simulink model "Diagrama_fotovoltaica_pk"  (R2019a)
settings: Solver=VariableStepAuto  StartTime=0.0  StopTime=24.0  RelTol=1e-3
values from neighbouring files (symbols this model uses):
  T_muestreo = 1    [Inicializacion_datos_distrito_personalizado.m]    (also in Inicializacion_datos_invernadero_tradicional.m; Inicializacion_datos_microred.m; Inicializacion_datos_nanofiltracion.m; Inicializacion_datos_oficinas.m)
libraries: Libreria x2
settings Model: Creator=Usuario  LastModifiedBy=Usuario

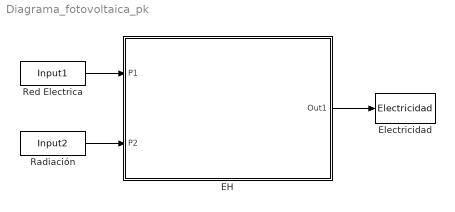
== system Diagrama_fotovoltaica_pk ==
  EH : Subsystem
  Electricidad : ToWorkspace  VariableName=Electricidad  SaveFormat=Timeseries  SampleTime=T_muestreo
  Radiación : FromWorkspace  VariableName=Input2  SampleTime=0
  Red Electrica : FromWorkspace  VariableName=Input1  SampleTime=0
  wires:
  Red Electrica/1 -> EH/1(P1)
  Radiación/1 -> EH/2(P2)
  EH/1(Out1) -> Electricidad/1

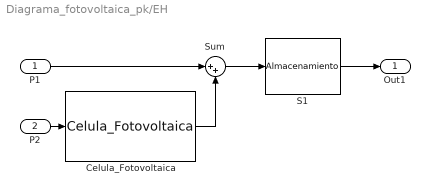
== system Diagrama_fotovoltaica_pk/EH ==
  P1 : Inport
  P2 : Inport  Port=2
  Celula_Fotovoltaica : Libreria/Celula_Fotovoltaica  efficiency=0.211  dispatch_factor=1  T_muestreo=T_muestreo  Max_in=1200  Max_out=2600
  S1 : Libreria/Almacenamiento  Up2=2000  Low2=500  r_c=1  Up=2000  Low=500  r_d=1  Up1=6000  Low1=500  almacenamiento_inicial=0  cpa=1  almacenamiento_on=on
      link override In1: SampleTime=1
      link override Qch: VariableName=Qchp1
      link override Qdis: VariableName=Qdisp1
      link override almacenamiento: VariableName=almacen1
      link override discrepancias_almacenamiento: VariableName=discrepancias_almacenamiento1
      link override ef: VariableName=Ech1
      link override eff: VariableName=Edis1
  Sum : Sum  Inputs=|++
  Out1 : Outport
  wires:
  Sum/1 -> S1/1
  S1/1 -> Out1/1
  P2/1 -> Celula_Fotovoltaica/1
  P1/1 -> Sum/1
  Celula_Fotovoltaica/1 -> Sum/2
